simulink model "v_0"  (R2017a)
settings: Solver=FixedStepDiscrete  StartTime=0.0  StopTime=10  FixedStep=0.001  RelTol=1e-3
settings Model: Creator=Vasilii  LastModifiedBy=Vasilii

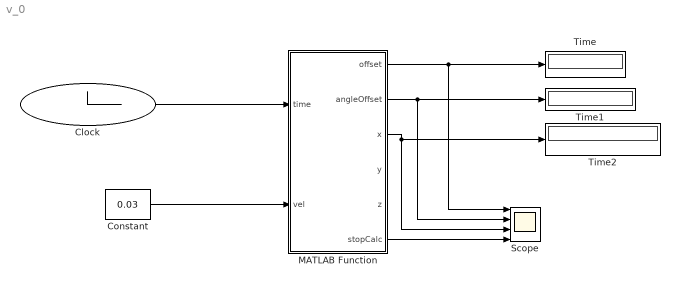
== system v_0 ==
  Clock : Clock
  Constant : Constant  Value=0.03
  MATLAB Function : MATLAB Function  TreatAsAtomicUnit=on
  Scope : Scope  NumInputPorts=4
  Time : Display
      settings: Decimation=4
  Time1 : Display
      settings: Decimation=4
  Time2 : Display
      settings: Decimation=4
  wires:
  Constant/1 -> MATLAB Function/2(vel)
  Clock/1 -> MATLAB Function/1(time)
  MATLAB Function/1(offset) -> Scope/1, Time/1
  MATLAB Function/6(stopCalc) -> Scope/4
  MATLAB Function/2(angleOffset) -> Time1/1, Scope/2
  MATLAB Function/3(x) -> Time2/1, Scope/3

== matlab function v_0/MATLAB Function ==
  data: time input; offset output; vel input; angleOffset output; x output; y output; z output; stopCalc output
function [offset,angleOffset,x,y,z,stopCalc] = fcn(time,vel)

[offset,angleOffset,x,y,z,stopCalc] = CalcFunction_v_0(time,vel);
